simulink model "vandevusse_EE"  (R2020b)
settings: Solver=ode45  StartTime=0.0  StopTime=0.4  MaxStep=1e-3  MinStep=1e-4  RelTol=1e-3
values from neighbouring files (symbols this model uses):
  x_ss = fsolve(@(x) model_vandevusse(0,x,u,p,d),x0,options)    [RGA_vandevusse.m]    (also in Van_de_vusse.m; Van_de_vusse_SS.m)
libraries: cstblocks x4
settings Model: Creator=Gustavo Caldas  LastModifiedBy=Gustavo Caldas

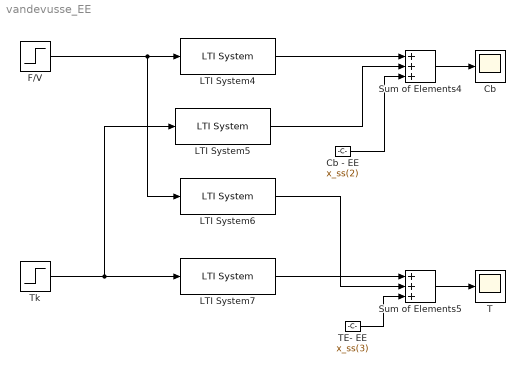
== system vandevusse_EE ==
  Cb : Scope
  Cb - EE : Constant  Value=x_ss(2)
  F/V : Step  Time=0  SampleTime=0
  LTI System4 : cstblocks/LTI System  sys=tf11  IC=[]
  LTI System5 : cstblocks/LTI System  sys=tf12  IC=[]
  LTI System6 : cstblocks/LTI System  sys=tf21  IC=[]
  LTI System7 : cstblocks/LTI System  sys=tf22  IC=[]
  Sum of Elements4 : Sum  Inputs=+++
  Sum of Elements5 : Sum  Inputs=+++
  T : Scope
  TE- EE : Constant  Value=x_ss(3)
  Tk : Step  Time=0  After=0  SampleTime=0
  wires:
  LTI System6/1 -> Sum of Elements5/2
  LTI System5/1 -> Sum of Elements4/2
  Sum of Elements5/1 -> T/1
  LTI System7/1 -> Sum of Elements5/1
  Tk/1 -> LTI System5/1, LTI System7/1
  Sum of Elements4/1 -> Cb/1
  F/V/1 -> LTI System6/1, LTI System4/1
  LTI System4/1 -> Sum of Elements4/1
  Cb - EE/1 -> Sum of Elements4/3
  TE- EE/1 -> Sum of Elements5/3
